simulink model "FIM"  (R2018b)
settings: Solver=ode8  StartTime=0.0  StopTime=0.2  RelTol=1e-3
undefined symbols (not defined in the file): Cout_c, Cout_r, Cvh_c, Cvh_r, dellay_f2, DiscIntNeverNeededParam, discret, f, L1_l, L1_r, Lvh_l, Lvh_r, R_out, Uout, Uvh
libraries: powerlib x18, powerlib_meascontrol x4, simulink x2, simulink_extras x2
settings Model: Creator=Anton  LastModifiedBy=VID Company
settings SFSimCC: SimUseLocalCustomCode=off
settings RTWCC: RTWUseLocalCustomCode=off
settings CodeAppCC: StateflowObjectComments=on
settings SimscapeCC: SimscapeNormalizeSystem=off

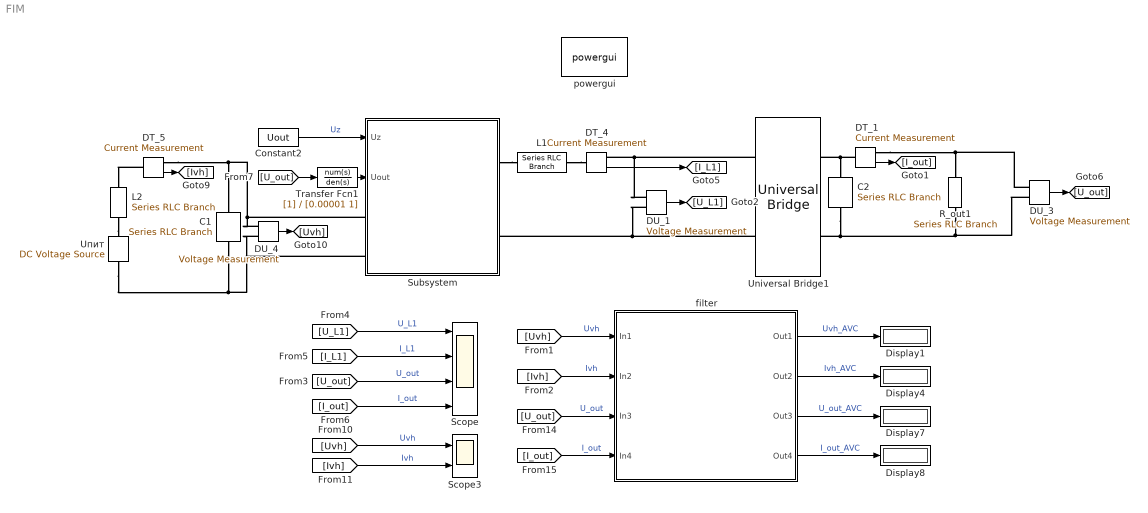
== system FIM ==
  C1 : powerlib/Elements/Series RLC Branch  LConnTagsString=__new0  RConnTagsString=__new0  BranchType=RC  Resistance=Cvh_r  Inductance=1e-3  SetiL0=off  InitialCurrent=0  Capacitance=Cvh_c  Setx0=on  InitialVoltage=Uvh  Measurements=Branch voltage
      settings: SourceProductName=Simscape Electrical
  C2 : powerlib/Elements/Series RLC Branch  LConnTagsString=__new0  RConnTagsString=__new0  BranchType=RC  Resistance=Cout_r  Inductance=1e-3  SetiL0=off  InitialCurrent=0  Capacitance=Cout_c  Setx0=on  InitialVoltage=0  Measurements=Branch voltage
      settings: SourceProductName=Simscape Electrical
  Constant2 : Constant  Value=Uout
  DT_1 : powerlib/Measurements/Current Measurement  PhasorSimulation=off  OutputType=Complex  PSBequivalent=0
      settings: SourceProductName=Simscape Electrical
  DT_4 : powerlib/Measurements/Current Measurement  PhasorSimulation=off  OutputType=Complex  PSBequivalent=0
      settings: SourceProductName=Simscape Electrical
  DT_5 : powerlib/Measurements/Current Measurement  PhasorSimulation=off  OutputType=Complex  PSBequivalent=0
      settings: SourceProductName=Simscape Electrical
  DU_1 : powerlib/Measurements/Voltage Measurement  PhasorSimulation=off  OutputType=Complex  PSBequivalent=0
      settings: SourceProductName=Simscape Electrical
  DU_3 : powerlib/Measurements/Voltage Measurement  PhasorSimulation=off  OutputType=Complex  PSBequivalent=0
      settings: SourceProductName=Simscape Electrical
  DU_4 : powerlib/Measurements/Voltage Measurement  PhasorSimulation=off  OutputType=Complex  PSBequivalent=0
      settings: SourceProductName=Simscape Electrical
  Display{1,4,7..8} (4 alike) : Display
  L1 : powerlib/Elements/Series RLC Branch  LConnTagsString=__new0  RConnTagsString=__new0  BranchType=RL  Resistance=L1_r  Inductance=L1_l  SetiL0=off  InitialCurrent=0  Capacitance=1e-6  Setx0=off  InitialVoltage=0  Measurements=None
      settings: SourceProductName=Simscape Electrical
  L2 : powerlib/Elements/Series RLC Branch  LConnTagsString=__new0  RConnTagsString=__new0  BranchType=RL  Resistance=Lvh_r  Inductance=Lvh_l  SetiL0=off  InitialCurrent=0  Capacitance=1e-6  Setx0=off  InitialVoltage=0  Measurements=None
      settings: SourceProductName=Simscape Electrical
  R_out1 : powerlib/Elements/Series RLC Branch  LConnTagsString=__new0  RConnTagsString=__new0  BranchType=R  Resistance=R_out  Inductance=1e-3  SetiL0=off  InitialCurrent=0  Capacitance=1e-6  Setx0=off  InitialVoltage=0  Measurements=None
      settings: SourceProductName=Simscape Electrical
  Scope : Scope  NumInputPorts=4
  Scope3 : Scope  NumInputPorts=2
  Subsystem : Subsystem
  Transfer Fcn1 : TransferFcn  Denominator=[0.00001 1]
  Universal Bridge1 : powerlib/Power Electronics/Universal Bridge  Arms=2  SnubberResistance=1e5  SnubberCapacitance=inf  Device=Diodes  Ron=3e-3  Lon=0  ForwardVoltages="[  0  0  ]"  ForwardVoltage=1  GTOparameters=[ 10e-6 , 20e-6 ]  IGBTparameters=[ 1e-6 , 2e-6 ]  Measurements=None  Measurements_2=None  converterType=Rectifier
  Uпит : powerlib/Electrical Sources/DC Voltage Source  Amplitude=Uvh  Measurements=None
      settings: SourceProductName=Simscape Electrical
  filter : Subsystem
  powergui : powerlib/powergui  Priority=1  SimulationMode=Discrete  SampleTime=discret  frequency=60  Iterations=50  frequencyindice=0  Pbase=100e6  ErrMax=1e-4  UnitsV=kV  UnitsW=MW  buscounter=0  FunctionMessages=off  echomessages=off  EnableUseOfTLC=off  CurrentSourceSwitches=off  DisableSnubberDevices=off  DisableRonSwitches=off  DisableVfSwitches=off  DisplayEquations=off  SolverType=Tustin/Backward Euler (TBE)  Interpol=off  ExternalGateDelay=off  methode=off  Ts=100  x0status=blocks  SPID=off  SwTol=0  HookPort=off  RestoreLinks=warning  ResistiveCurrentMeasurement=off  Frange=[0:2:500]  Ylog=off  Xlog=on  ShowGrid=off  save=off  variable=ZData  structure=0  ZoomFFT=off  StartTime=0.0  cycles=1  DisplayStyle=1  fundamental=60  FreqAxis=off  MaxFrequency=1000  frequencyindicesteady=1  RmsSteady=1  display=off
  wires:
  DT_4/1 -> [I_L1]
  DU_3/1 -> [U_out]
  [U_L1] -> Scope/1  "U_L1"
  [I_L1] -> Scope/2  "I_L1"
  DT_5/1 -> [Ivh]
  DU_4/1 -> [Uvh]
  [Ivh] -> Scope3/2  "Ivh"
  [Uvh] -> Scope3/1  "Uvh"
  [U_out] -> filter/3(In3)  "U_out"
  [I_out] -> filter/4(In4)  "I_out"
  [Uvh] -> filter/1(In1)  "Uvh"
  [Ivh] -> filter/2(In2)  "Ivh"
  filter/1(Out1) -> Display1/1  "Uvh_AVC"
  filter/2(Out2) -> Display4/1  "Ivh_AVC"
  filter/3(Out3) -> Display7/1  "U_out_AVC"
  filter/4(Out4) -> Display8/1  "I_out_AVC"
  [U_out] -> Scope/3  "U_out"
  [I_out] -> Scope/4  "I_out"
  DT_1/1 -> [I_out]
  DU_1/1 -> [U_L1]
  [U_out] -> Transfer Fcn1/1
  Transfer Fcn1/1 -> Subsystem/2(Uout)
  Constant2/1 -> Subsystem/1(Uz)  "Uz"
  connections:
  DU_4/LConn1 -- DT_5/RConn1 -- C1/LConn1 -- Subsystem/LConn1
  L2/LConn1 -- Uпит/RConn1
  DT_5/LConn1 -- L2/RConn1
  C1/RConn1 -- DU_4/LConn2 -- Subsystem/LConn2 -- Uпит/LConn1
  Subsystem/RConn1 -- L1/LConn1
  L1/RConn1 -- DT_4/LConn1
  Universal Bridge1/LConn1 -- DU_1/LConn1 -- DT_4/RConn1
  Universal Bridge1/LConn2 -- DU_1/LConn2 -- Subsystem/RConn2
  DT_1/LConn1 -- C2/LConn1 -- Universal Bridge1/RConn1
  DU_3/LConn1 -- R_out1/LConn1 -- DT_1/RConn1
  R_out1/RConn1 -- Universal Bridge1/RConn2 -- C2/RConn1 -- DU_3/LConn2

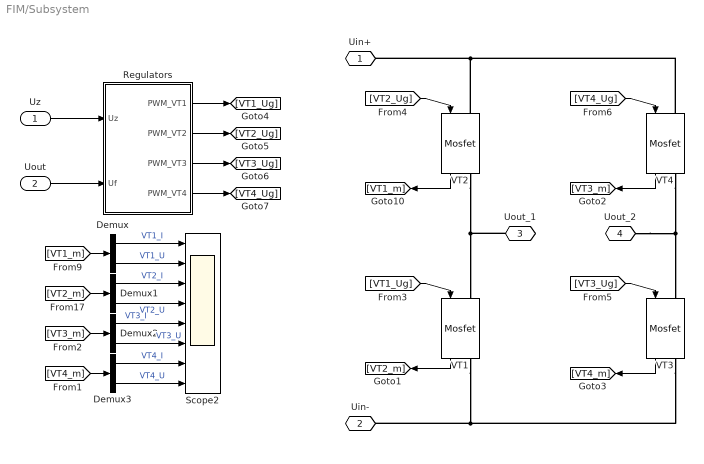
== system FIM/Subsystem ==
  Uz : Inport
  Uout : Inport  Port=2
  Demux{,1..3} (4 alike) : Demux  Outputs=2
  Regulators : Subsystem
  Scope2 : Scope  NumInputPorts=8
  VT{1..4} (4 alike) : powerlib/Power Electronics/Mosfet  Ron=10e-3  Lon=inf  Rd=10e-3  Vfd=1  IC=0  Rs=1e5  Cs=inf  Measurements=on
      settings: SourceProductName=Simscape Electrical
  Uin+ : PMIOPort  Side=Left
  Uin- : PMIOPort  Port=2  Side=Left
  Uout_1 : PMIOPort  Port=3  Side=Right
  Uout_2 : PMIOPort  Port=4  Side=Right
  wires:
  [VT2_m] -> Demux1/1
  Demux1/2 -> Scope2/4  "VT2_U"
  Demux/1 -> Scope2/1  "VT1_I"
  Demux/2 -> Scope2/2  "VT1_U"
  Demux1/1 -> Scope2/3  "VT2_I"
  [VT1_m] -> Demux/1
  VT2/1 -> [VT1_m]
  VT1/1 -> [VT2_m]
  VT4/1 -> [VT3_m]
  VT3/1 -> [VT4_m]
  [VT3_m] -> Demux2/1
  Demux3/1 -> Scope2/7  "VT4_I"
  Demux2/2 -> Scope2/6  "VT3_U"
  Demux3/2 -> Scope2/8  "VT4_U"
  Demux2/1 -> Scope2/5  "VT3_I"
  [VT4_m] -> Demux3/1
  Regulators/1(PWM_VT1) -> [VT1_Ug]
  Regulators/2(PWM_VT2) -> [VT2_Ug]
  Regulators/3(PWM_VT3) -> [VT3_Ug]
  Regulators/4(PWM_VT4) -> [VT4_Ug]
  [VT1_Ug] -> VT1/1
  [VT2_Ug] -> VT2/1
  [VT3_Ug] -> VT3/1
  [VT4_Ug] -> VT4/1
  Uout/1 -> Regulators/2(Uf)
  Uz/1 -> Regulators/1(Uz)
  connections:
  VT2/RConn1 -- Uout_1/RConn1 -- VT1/LConn1
  VT2/LConn1 -- VT4/LConn1 -- Uin+/RConn1
  VT1/RConn1 -- VT3/RConn1 -- Uin-/RConn1
  VT4/RConn1 -- Uout_2/RConn1 -- VT3/LConn1

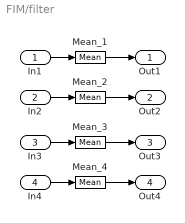
== system FIM/filter ==
  In1 : Inport
  In2 : Inport  Port=2
  In3 : Inport  Port=3
  In4 : Inport  Port=4
  Mean_{1..4} (4 alike) : powerlib_meascontrol/Measurements/Mean  Freq=100  Vinit=0  Ts=0
  Out1 : Outport
  Out2 : Outport  Port=2
  Out3 : Outport  Port=3
  Out4 : Outport  Port=4
  wires:
  In1/1 -> Mean_1/1
  In2/1 -> Mean_2/1
  In3/1 -> Mean_3/1
  In4/1 -> Mean_4/1
  Mean_1/1 -> Out1/1
  Mean_2/1 -> Out2/1
  Mean_3/1 -> Out3/1
  Mean_4/1 -> Out4/1

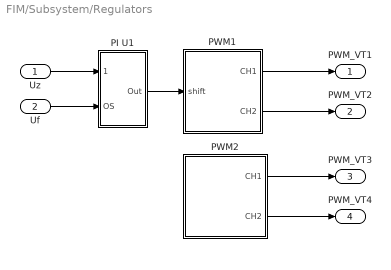
== system FIM/Subsystem/Regulators ==
  Uz : Inport
  Uf : Inport  Port=2
  PI U1 : Subsystem
  PWM1 : Subsystem
  PWM2 : Subsystem
  PWM_VT1 : Outport
  PWM_VT2 : Outport  Port=2
  PWM_VT3 : Outport  Port=3
  PWM_VT4 : Outport  Port=4
  wires:
  PI U1/1(Out) -> PWM1/1(shift)
  Uz/1 -> PI U1/1(Zad)
  Uf/1 -> PI U1/2(OS)
  PWM1/1(CH1) -> PWM_VT1/1
  PWM1/2(CH2) -> PWM_VT2/1
  PWM2/1(CH1) -> PWM_VT3/1
  PWM2/2(CH2) -> PWM_VT4/1

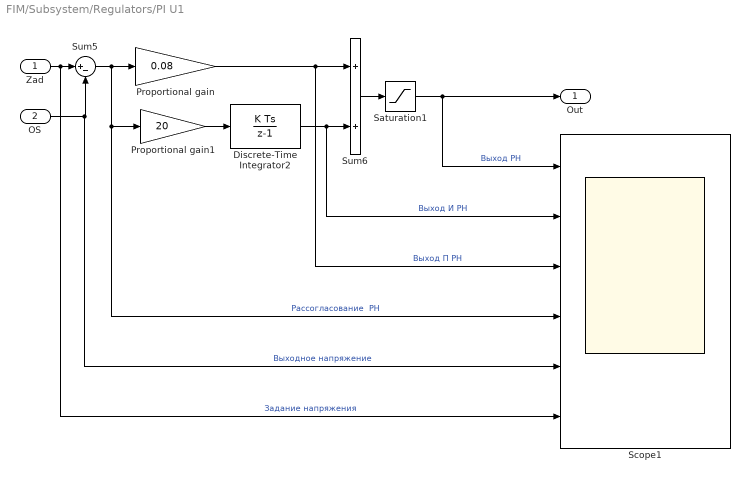
== system FIM/Subsystem/Regulators/PI U1 ==
  Zad : Inport
  OS : Inport  Port=2
  Discrete-Time Integrator2 : DiscreteIntegrator  SampleTime=-1  LimitOutput=on  UpperSaturationLimit=120  LowerSaturationLimit=0  ICPrevOutput=DiscIntNeverNeededParam  ICPrevScaledInput=DiscIntNeverNeededParam
  Proportional gain : Gain  Gain=0.08  SaturateOnIntegerOverflow=on  OutDataTypeStr=Inherit: Same as input  ParamDataTypeStr=Inherit: Same as input
  Proportional gain1 : Gain  Gain=20  SaturateOnIntegerOverflow=on  OutDataTypeStr=Inherit: Same as input  ParamDataTypeStr=Inherit: Same as input
  Saturation1 : Saturate  UpperLimit=120  LowerLimit=0
  Scope1 : Scope  NumInputPorts=6
  Sum5 : Sum  Inputs=|+-  SaturateOnIntegerOverflow=on  InputSameDT=on  OutDataTypeStr=Inherit: Same as first input
  Sum6 : Sum  SaturateOnIntegerOverflow=on  InputSameDT=on  OutDataTypeStr=Inherit: Same as first input
  Out : Outport
  wires:
  Proportional gain/1 -> Scope1/3, Sum6/1  "Выход П РН"
  Discrete-Time Integrator2/1 -> Sum6/2, Scope1/2  "Выход И РН"
  OS/1 -> Scope1/5, Sum5/2  "Выходное напряжение"
  Zad/1 -> Scope1/6, Sum5/1  "Задание напряжения"
  Sum5/1 -> Proportional gain1/1, Scope1/4, Proportional gain/1  "Рассогласование  РН"
  Sum6/1 -> Saturation1/1
  Saturation1/1 -> Out/1, Scope1/1  "Выход РН"
  Proportional gain1/1 -> Discrete-Time Integrator2/1

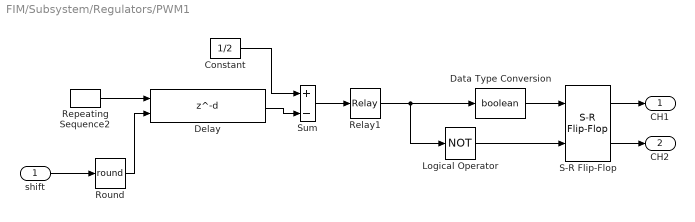
== system FIM/Subsystem/Regulators/PWM1 ==
  shift : Inport
  Constant : Constant  Value=1/2
  Data Type Conversion : DataTypeConversion  OutDataTypeStr=boolean
  Delay : Delay  DelayLengthSource=Input port  DelayLength=dellay_f2  DelayLengthUpperLimit=2000
      settings: InputPortMap=u0,p1
  Logical Operator : Logic  Operator=NOT  AllPortsSameDT=off  OutDataTypeStr=boolean
  Relay1 : Relay  OnSwitchValue=0.01  OffSwitchValue=-0.01
  Repeating Sequence2 : simulink/Sources/Repeating Sequence  rep_seq_t="[0  (1/(2*f)) (1/f)]"  rep_seq_y=[0 1 0]
  Round : Rounding  Operator=round
  S-R Flip-Flop : simulink_extras/Flip Flops/S-R Flip-Flop  initial_condition=0
  Sum : Sum  Inputs=+-
  CH1 : Outport
  CH2 : Outport  Port=2
  wires:
  S-R Flip-Flop/1 -> CH1/1
  Data Type Conversion/1 -> S-R Flip-Flop/1
  Logical Operator/1 -> S-R Flip-Flop/2
  Relay1/1 -> Logical Operator/1, Data Type Conversion/1
  Sum/1 -> Relay1/1
  S-R Flip-Flop/2 -> CH2/1
  Constant/1 -> Sum/1
  Repeating Sequence2/1 -> Delay/1
  Delay/1 -> Sum/2
  shift/1 -> Round/1
  Round/1 -> Delay/2

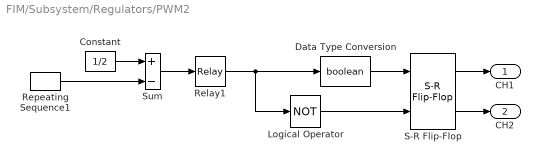
== system FIM/Subsystem/Regulators/PWM2 ==
  Constant : Constant  Value=1/2
  Data Type Conversion : DataTypeConversion  OutDataTypeStr=boolean
  Logical Operator : Logic  Operator=NOT  AllPortsSameDT=off  OutDataTypeStr=boolean
  Relay1 : Relay  OnSwitchValue=0.01  OffSwitchValue=-0.01
  Repeating Sequence1 : simulink/Sources/Repeating Sequence  rep_seq_t="[0  (1/(2*f)) (1/f)]"  rep_seq_y=[0 1 0]
  S-R Flip-Flop : simulink_extras/Flip Flops/S-R Flip-Flop  initial_condition=0
  Sum : Sum  Inputs=+-
  CH1 : Outport
  CH2 : Outport  Port=2
  wires:
  S-R Flip-Flop/1 -> CH1/1
  Data Type Conversion/1 -> S-R Flip-Flop/1
  Logical Operator/1 -> S-R Flip-Flop/2
  Relay1/1 -> Logical Operator/1, Data Type Conversion/1
  Sum/1 -> Relay1/1
  S-R Flip-Flop/2 -> CH2/1
  Repeating Sequence1/1 -> Sum/2
  Constant/1 -> Sum/1
